simulink model "RCAMSimulation"  (R2016b)
settings: Solver=VariableStepAuto  StartTime=0.0  StopTime=TF  RelTol=1e-3
values from neighbouring files (symbols this model uses):
  u1max = 25*pi/180    (= 0.436332312999)    [Initialize.m]
  u1min = -25*pi/180    (= -0.436332312999)    [Initialize.m]
  u2max = 10*pi/180    (= 0.174532925199)    [Initialize.m]
  u2min = -25*pi/180    (= -0.436332312999)    [Initialize.m]
  u3max = 30*pi/180    (= 0.523598775598)    [Initialize.m]
  u3min = -30*pi/180    (= -0.523598775598)    [Initialize.m]
  u4max = 10*pi/180    (= 0.174532925199)    [Initialize.m]
  u4min = 0*pi/180    (= 0)    [Initialize.m]
  u5max = 10*pi/180    (= 0.174532925199)    [Initialize.m]
  u5min = 0*pi/180    (= 0)    [Initialize.m]
  x0 = [85 ... (first row only)    [Initialize.m]
undefined symbols (not defined in the file or in its folder): RCAM_model
settings Model: Creator=13911  LastModifiedBy=13911

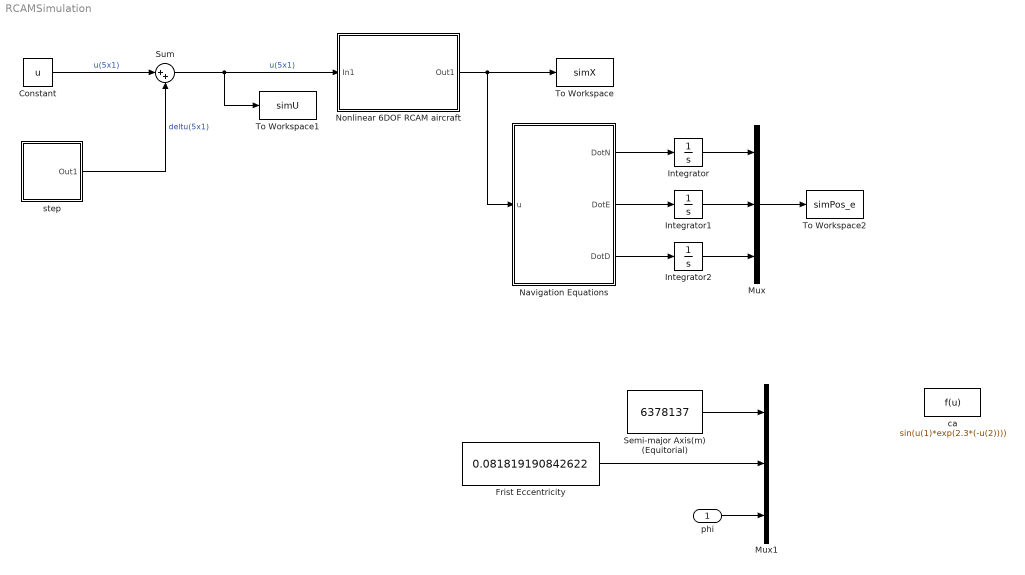
== system RCAMSimulation ==
  phi : Inport
  Constant : Constant  Value=u
  Frist Eccentricity : Constant  Value=0.081819190842622
  Integrator : Integrator
  Integrator1 : Integrator
  Integrator2 : Integrator
  Mux : Mux  Inputs=3
  Mux1 : Mux  Inputs=3
  Navigation Equations : MATLAB Function  TreatAsAtomicUnit=on
  Nonlinear 6DOF RCAM aircraft : Subsystem
  Semi-major Axis(m) (Equitorial) : Constant  Value=6378137
  Sum : Sum  Inputs=|++
  To Workspace : ToWorkspace  VariableName=simX  SaveFormat=Timeseries  SampleTime=-1
  To Workspace1 : ToWorkspace  VariableName=simU  SaveFormat=Timeseries  SampleTime=-1
  To Workspace2 : ToWorkspace  VariableName=simPos_e  SaveFormat=Timeseries  SampleTime=-1
  ca : Fcn  Expr=sin(u(1)*exp(2.3*(-u(2))))
  step : Subsystem
  wires:
  Sum/1 -> Nonlinear 6DOF RCAM aircraft/1(In1), To Workspace1/1  "u(5x1)"
  Nonlinear 6DOF RCAM aircraft/1(Out1) -> Navigation Equations/1(u), To Workspace/1
  Constant/1 -> Sum/1  "u(5x1)"
  step/1(Out1) -> Sum/2  "deltu(5x1)"
  Navigation Equations/1(DotN) -> Integrator/1
  Navigation Equations/2(DotE) -> Integrator1/1
  Navigation Equations/3(DotD) -> Integrator2/1
  Integrator2/1 -> Mux/3
  Integrator1/1 -> Mux/2
  Integrator/1 -> Mux/1
  Mux/1 -> To Workspace2/1
  Semi-major Axis(m) (Equitorial)/1 -> Mux1/1
  Frist Eccentricity/1 -> Mux1/2
  phi/1 -> Mux1/3

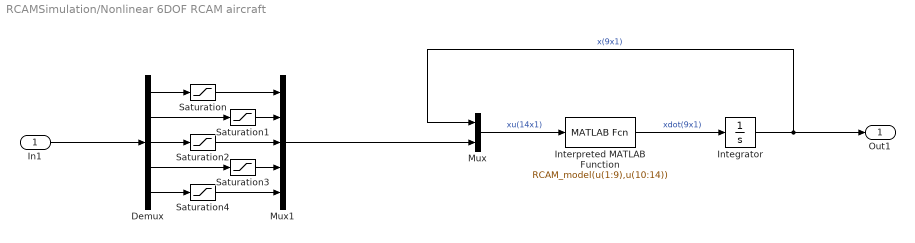
== system RCAMSimulation/Nonlinear 6DOF RCAM aircraft ==
  In1 : Inport
  Demux : Demux  Outputs=5
  Integrator : Integrator  InitialCondition=x0
  Interpreted MATLAB Function : MATLABFcn  MATLABFcn=RCAM_model(u(1:9),u(10:14))
  Mux : Mux  Inputs=2
  Mux1 : Mux  Inputs=5
  Saturation : Saturate  UpperLimit=u1max  LowerLimit=u1min
  Saturation1 : Saturate  UpperLimit=u2max  LowerLimit=u2min
  Saturation2 : Saturate  UpperLimit=u3max  LowerLimit=u3min
  Saturation3 : Saturate  UpperLimit=u4max  LowerLimit=u4min
  Saturation4 : Saturate  UpperLimit=u5max  LowerLimit=u5min
  Out1 : Outport
  wires:
  Mux/1 -> Interpreted MATLAB Function/1  "xu(14x1)"
  Interpreted MATLAB Function/1 -> Integrator/1  "xdot(9x1)"
  Integrator/1 -> Out1/1, Mux/1  "x(9x1)"
  In1/1 -> Demux/1
  Demux/1 -> Saturation/1
  Demux/2 -> Saturation1/1
  Demux/3 -> Saturation2/1
  Demux/4 -> Saturation3/1
  Demux/5 -> Saturation4/1
  Mux1/1 -> Mux/2
  Saturation/1 -> Mux1/1
  Saturation1/1 -> Mux1/2
  Saturation2/1 -> Mux1/3
  Saturation3/1 -> Mux1/4
  Saturation4/1 -> Mux1/5

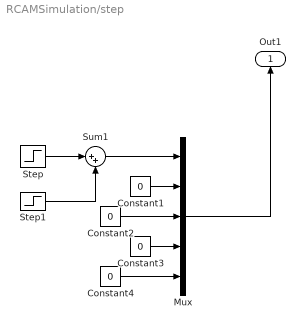
== system RCAMSimulation/step ==
  Constant{1..4} (4 alike) : Constant  Value=0
  Mux : Mux  Inputs=5
  Step : Step  Time=30  SampleTime=0
  Step1 : Step  Time=32  After=-1  SampleTime=0
  Sum1 : Sum  Inputs=|++
  Out1 : Outport
  wires:
  Step1/1 -> Sum1/2
  Sum1/1 -> Mux/1
  Step/1 -> Sum1/1
  Mux/1 -> Out1/1
  Constant1/1 -> Mux/2
  Constant4/1 -> Mux/5
  Constant3/1 -> Mux/4
  Constant2/1 -> Mux/3

== matlab function RCAMSimulation/Navigation Equations ==
  data: u input; DotN output; DotE output; DotD output
function [DotN,DotE,DotD] = fcn(u)
x1 = u(1);
x2 = u(2);
x3 = u(3);
x4 = u(4);
x5 = u(5);
x6 = u(6);
x7 = u(7);
x8 = u(8);
x9 = u(9);




c1v = [cos(x9),sin(x9),0;-sin(x9),cos(x9),0;0,0,1];
c21 = [cos(x8),0,-sin(x8);0,1,0;sin(x8),0,cos(x8)];
cb2 = [1,0,0;0,cos(x7),sin(x7);0,-sin(x7),cos(x7)];

cbv = cb2*c21*c1v;
cvb = cbv';
V_b = [x1,x2,x3]';
V_e = cvb*V_b ;
DotN= V_e(1);
DotE= V_e(2);
DotD= V_e(3);
